simulink model "all_in_one"  (R2015a)
settings: Solver=ode45  StartTime=0.0  StopTime=10.0  RelTol=1e-3
settings Model: CovSFcnEnable=off  Creator=qiji  LastModifiedBy=qiji
settings DebuggingCC: UnderspecifiedInitializationDetection=Classic  MergeDetectMultiDrivingBlocksExec=none  SolverPrmCheckMsg=warning

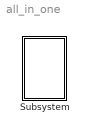
== system all_in_one ==
  Subsystem : Subsystem

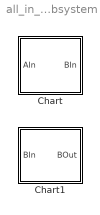
== system all_in_one/Subsystem ==
  Chart : Stateflow chart  TreatAsAtomicUnit=on
  Chart1 : Stateflow chart  TreatAsAtomicUnit=on

== stateflow chart all_in_one/Subsystem/Chart ==
  state A
    en:
    AOut = 0;
  state B
    en:
    AOut = 1;
  A -> B : [AIn == 1]
  (default) -> A
  B -> A : [AIn==1]
  data: AIn input double; BIn output double
  data AIn settings: description=in

== stateflow chart all_in_one/Subsystem/Chart1 ==
  state A
    du:
    BOut = BIn
  (default) -> A
  data: BOut output double; BIn input double
  data BOut settings: description=out
